simulink model "satellite_behaviour"  (Simulink 6.3)
settings: Solver=ode45  StartTime=0.0  StopTime=1000  RelTol=1e-3
libraries: components_lib x6, simulink x1
settings Model: Creator=krage  LastModifiedBy=mnkr02  ExtModeAutoUpdateStatusClock=off  StrictBusMsg=None

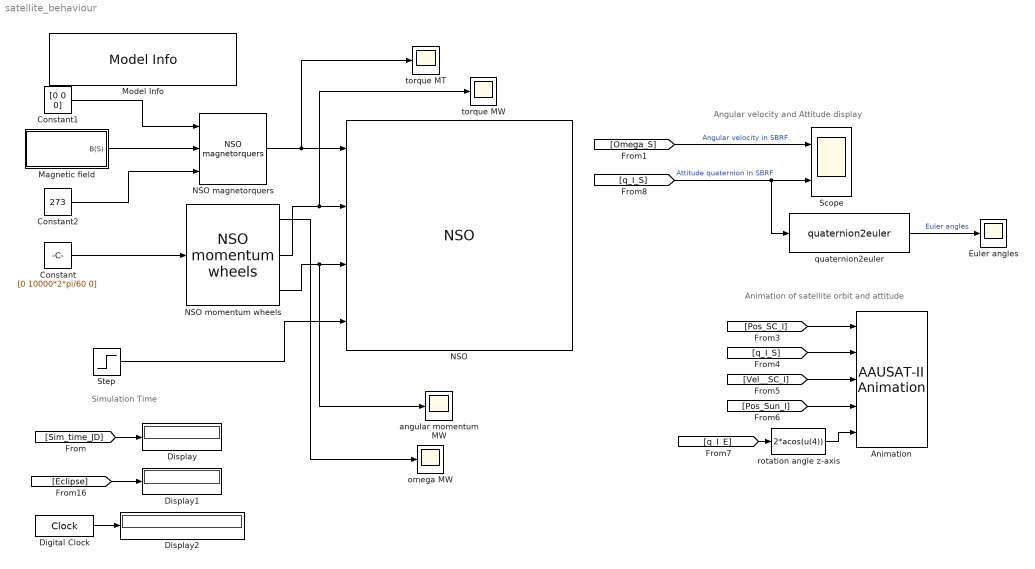
== system satellite_behaviour ==
  note: Simulation Time
  note: Angular velocity and Attitude display
  note: Animation of satellite orbit and attitude
  Animation : components_lib/Other model utilities/AAUSAT-II Animation  u1=[-20000000 20000000 -20000000 20000000 -20000000 20000000]  u2=50  u3=1000000  u20=on  u18=15  u4=6378000  u11=80  u12=on  u13='earth280.jpg'  u17=180  u5=Fixed position  u6=[70000000 70000000 70000000]  u7=8  u9=off  u10=on  u16=off  u14=on  u15=on  u8=on  u19=off
  Constant : Constant  Value=[0 10000*2*pi/60 0]
  Constant1 : Constant  Value=[0 0 0]
  Constant2 : Constant  Value=273
  Digital Clock : DigitalClock
  Display : Display
  Display1 : Display
  Display2 : Display
  Euler angles : Scope
      settings: YMin=-3.5  YMax=3.5
  Magnetic field : Subsystem
  Model Info : simulink/Model-Wide Utilities/Model Info  InitialBlockCM=None  BlockCM=None  Frame=on  DisplayStringWithTags=|  HorizontalTextAlignment=Center  LeftAlignmentValue=0.5  SourceBlockDiagram=satellite_behaviour  TagMaxNumber=20
      | sun to eclipse : 2452315.560376
      | 32 sec. before : 2452315.56
      | eclipse to sun : 2452315.513363
  NSO : components_lib/NSO  Tag=AAUSAT-II Model  Description=AAUSAT-II Model  r_com_s=[0.05 0.05 0.15]  sat_temp_start=0  r_com_s_deployed=[0.05 0.05 0.125]  mass_sc=3  Dim=[0.1 0.1 0.3]  inertia_c=[25 25 5]/1e3  inertia_d=[42.3 42.3 28.4]/1e3  init_jd=2452315.56  q_s_c=[0 0 0 1]  q_init_s_i=[sqrt(0.5) 0 0 sqrt(0.5)]  w_init_s=[0.1 0.1 0.1]*0  Cd=2  rho=9.25e-13  enable_sensor_emulation=off  alb_emu_enabled=off  enable_dist=off
  NSO magnetorquers : components_lib/Actuator Emulation/NSO magnetorquers
  NSO momentum wheels : components_lib/Actuator Emulation/NSO momentum wheels  w_mw_i=[1078.6 1078.6 1078.6] *0.5
  Scope : Scope  NumInputPorts=2
      settings: YMin=-5~-5  YMax=5~5
  Step : Step  Time=500  SampleTime=0
  angular momentum MW : Scope
      settings: YMin=0  YMax=0.0045  SaveName=ScopeData4
  omega MW : Scope
      settings: YMin=0  YMax=1100  SaveName=ScopeData5
  quaternion2euler : components_lib/Math utilities/Quaternion operations/quaternion2euler
  rotation angle z-axis : MATLABFcn  MATLABFcn=2*acos(u(4))
  torque MT : Scope
      settings: YMin=-1  YMax=1  SaveName=ScopeData2
  torque MW : Scope
      settings: YMin=-0.0045  YMax=0.003  SaveName=ScopeData3
  wires:
  [Omega_S] -> Scope/1  "Angular velocity in SBRF"
  [q_I_S] -> quaternion2euler/1, Scope/2  "Attitude quaternion in SBRF"
  quaternion2euler/1 -> Euler angles/1  "Euler angles"
  [Sim_time_JD] -> Display/1
  [Eclipse] -> Display1/1
  [q_I_E] -> rotation angle z-axis/1
  [Pos_SC_I] -> Animation/1
  [q_I_S] -> Animation/2
  [Vel__SC_I] -> Animation/3
  [Pos_Sun_I] -> Animation/4
  rotation angle z-axis/1 -> Animation/5
  Digital Clock/1 -> Display2/1
  NSO magnetorquers/1 -> NSO/1, torque MT/1
  NSO momentum wheels/3 -> NSO/3, angular momentum MW/1
  NSO momentum wheels/2 -> NSO/2, torque MW/1
  Magnetic field/1(B(S)) -> NSO magnetorquers/2
  Constant/1 -> NSO momentum wheels/1
  Constant1/1 -> NSO magnetorquers/1
  Constant2/1 -> NSO magnetorquers/3
  NSO momentum wheels/1 -> omega MW/1
  Step/1 -> NSO/4

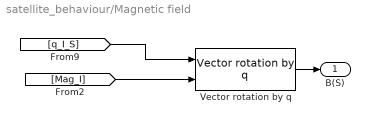
== system satellite_behaviour/Magnetic field ==
  Vector rotation by q : components_lib/Math utilities/Quaternion operations/Vector rotation by q
  B(S) : Outport
  wires:
  [q_I_S] -> Vector rotation by q/1
  [Mag_I] -> Vector rotation by q/2
  Vector rotation by q/1 -> B(S)/1
